simulink model "lump_model_v8"  (R2024b)
settings: Solver=FixedStepAuto  StartTime=0.0  StopTime=1079  FixedStep=0.001  RelTol=1e-3
model workspace (MAT data in the model file):
  A_busbar = 0.0015
  A_pack = 0.711626248
  C_nominal = 3
  I_max = 157.708978328
  P = 5
  S = 138
  SoC_initial = 0.78
  T_amb = 297.15
  W_max = 34
  busbar_CC_area = 0.000108
  busbar_Cp = 237
  busbar_length = 0.032
  busbar_mass = 0.01
  busbar_resistivity = 1.68e-08
  busbar_thermalcontact_resistance = 1
  cell_Cp = 1000
  cell_mass = 0.046
  h_busbar = 5
  h_pack = 5
(part 3 of 3)

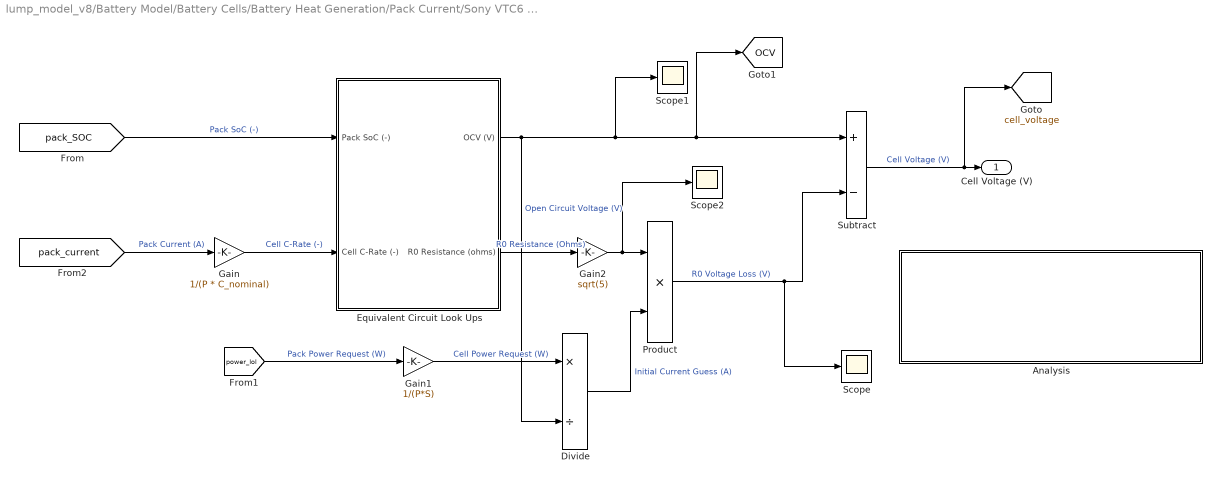
== system lump_model_v8/Battery Model/Battery Cells/Battery Heat Generation/Pack Current/Sony VTC6 Equivalent Circuit ==
  Analysis : Subsystem
  Divide : Product  Inputs=*/
  Equivalent Circuit Look Ups : Subsystem
  Gain : Gain  Gain=1/(P * C_nominal)
  Gain1 : Gain  Gain=1/(P*S)
  Gain2 : Gain  Gain=sqrt(5)
  Product : Product
  Scope : Scope
  Scope1 : Scope
  Scope2 : Scope
  Subtract : Sum  Inputs=+-
  Cell Voltage (V) : Outport
  tag scope: OCV=global, cell_voltage=global
  wires:
  [pack_SOC] -> Equivalent Circuit Look Ups/1(Pack SoC (-))  "Pack SoC (-)"
  Gain/1 -> Equivalent Circuit Look Ups/2(Cell C-Rate (-))  "Cell C-Rate (-)"
  Equivalent Circuit Look Ups/2(R0 Resistance (ohms)) -> Gain2/1  "R0 Resistance (Ohms)"
  Equivalent Circuit Look Ups/1(OCV (V)) -> Scope1/1, [OCV], Subtract/1, Divide/2  "Open Circuit Voltage (V)"
  Product/1 -> Scope/1, Subtract/2  "R0 Voltage Loss (V)"
  Subtract/1 -> [cell_voltage], Cell Voltage (V)/1  "Cell Voltage (V)"
  Divide/1 -> Product/2  "Initial Current Guess (A)"
  [power_lol] -> Gain1/1  "Pack Power Request (W)"
  Gain1/1 -> Divide/1  "Cell Power Request (W)"
  [pack_current] -> Gain/1  "Pack Current (A)"
  Gain2/1 -> Scope2/1, Product/1

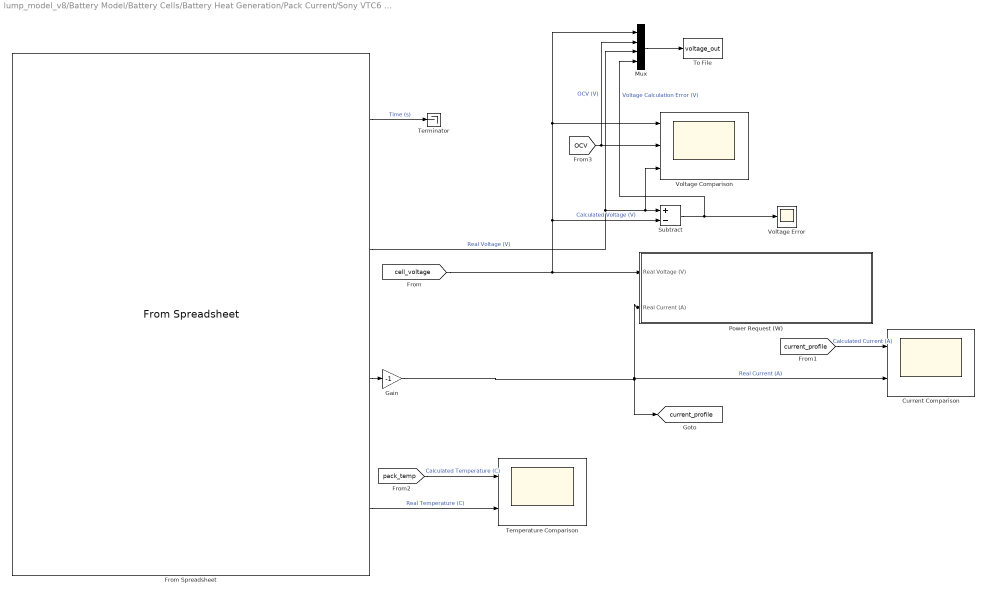
== system lump_model_v8/Battery Model/Battery Cells/Battery Heat Generation/Pack Current/Sony VTC6 Equivalent Circuit/Analysis ==
  Current Comparison : Scope  NumInputPorts=2
  From Spreadsheet : FromSpreadsheet  FileName=arbincomparisondata.xlsx  TreatFirstColumnAs=Data  SampleTime=0.003
  Gain : Gain  Gain=-1
  Mux : Mux
  Power Request (W) : Subsystem
  Subtract : Sum  Inputs=+-
  Temperature Comparison : Scope  NumInputPorts=2
  Terminator : Terminator
  To File : ToFile  Filename=voltage_out  MatrixName=voltage  SampleTime=0.01
  Voltage Comparison : Scope  NumInputPorts=3
  Voltage Error : Scope
  tag scope: current_profile=global
  wires:
  [cell_voltage] -> Power Request (W)/1(Real Voltage (V)), Subtract/2, Mux/1, Voltage Comparison/1  "Calculated Voltage (V)"
  [current_profile] -> Current Comparison/1  "Calculated Current (A)"
  [pack_temp] -> Temperature Comparison/1  "Calculated Temperature (C)"
  From Spreadsheet/2 -> Mux/3, Subtract/1, Voltage Comparison/3  "Real Voltage (V)"
  From Spreadsheet/3 -> Gain/1
  From Spreadsheet/4 -> Temperature Comparison/2  "Real Temperature (C)"
  From Spreadsheet/1 -> Terminator/1  "Time (s)"
  Gain/1 -> Current Comparison/2, Power Request (W)/2(Real Current (A)), [current_profile]  "Real Current (A)"
  Subtract/1 -> Mux/4, Voltage Error/1  "Voltage Calculation Error (V)"
  [OCV] -> Mux/2, Voltage Comparison/2  "OCV (V)"
  Mux/1 -> To File/1

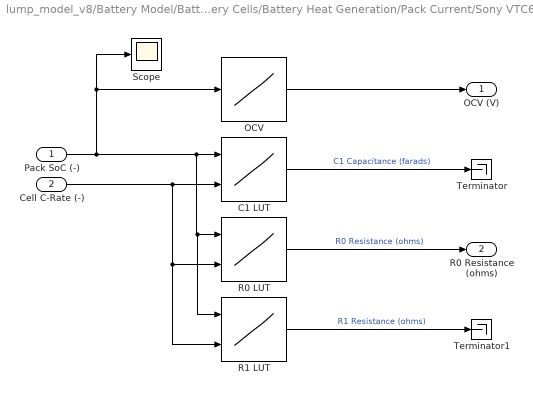
== system lump_model_v8/Battery Model/Battery Cells/Battery Heat Generation/Pack Current/Sony VTC6 Equivalent Circuit/Equivalent Circuit Look Ups ==
  Pack SoC (-) : Inport
  Cell C-Rate (-) : Inport  Port=2
  C1 LUT : Lookup_n-D  BreakpointsForDimension1=[0.1;0.2;0.3;0.4;0.5;0.6;0.7;0.8;0.9;1]  BreakpointsForDimension2=[-10;-5;-1;-0.333;0.333;1;2;3]  Table=[0.018906 0.021356 0.02305 0.022911 0.023301 0.023001 0.022654 0.019898;0.01868 0.020344 0.020909 0.020815 0.020944 0.020599 0.020712 0.017891;0.018453 0.019332 0.018859 0.023564 0.020028 0.019683 0.018901 0.017366;0.018226 0.019017 0.019644 0.020423 0.019635 0.019161 0.018682 0.01725;0.017999 0.018694 0.019687 0.020161 0.019897 0.01894 0.018442 0.01725;0.017916 0.018598 0.018989 0.01859 0.019505 0.018506 0.018289 0.017251;0.017743 0.018319 0.018291 0.022256 0.019767 0.018636 0.017788 0.017251;0.018183 0.018773 0.019295 0.021996 0.019898 0.019336 0.017286 0.017251;0.019549 0.020642 0.021608 0.025136 0.022253 0.020993 0.016785 0.017251;0.022703 0.024917 0.026536 0.026706 0.024609 0.02265 0.016283 0.017251]  ExtrapMethod=Clip  InternalRulePriority=Speed  RndMeth=Simplest
      settings: InputPortMap=u0,u1
  OCV : Lookup_n-D  NumberOfTableDimensions=1  BreakpointsForDimension1=[0.1;0.2;0.3;0.4;0.5;0.6;0.7;0.8;0.9;1]  BeginIndexSearchUsingPreviousIndexResult=on  Table=[3.227877;3.437376;3.537935;3.663634;3.755814;3.835423;3.940172;4.047017;4.097296;4.187904]  InternalRulePriority=Speed  RndMeth=Simplest
  R0 LUT : Lookup_n-D  BreakpointsForDimension1=[0.1;0.2;0.3;0.4;0.5;0.6;0.7;0.8;0.9;1]  BreakpointsForDimension2=[-10;-5;-1;-0.333;0.333;1;2;3]  Table=[0.018906 0.021356 0.02305 0.022911 0.023301 0.023001 0.022654 0.019898;0.01868 0.020344 0.020909 0.020815 0.020944 0.020599 0.020712 0.017891;0.018453 0.019332 0.018859 0.023564 0.020028 0.019683 0.018901 0.017366;0.018226 0.019017 0.019644 0.020423 0.019635 0.019161 0.018682 0.01725;0.017999 0.018694 0.019687 0.020161 0.019897 0.01894 0.018442 0.01725;0.017916 0.018598 0.018989 0.01859 0.019505 0.018506 0.018289 0.017251;0.017743 0.018319 0.018291 0.022256 0.019767 0.018636 0.017788 0.017251;0.018183 0.018773 0.019295 0.021996 0.019898 0.019336 0.017286 0.017251;0.019549 0.020642 0.021608 0.025136 0.022253 0.020993 0.016785 0.017251;0.022703 0.024917 0.026536 0.026706 0.024609 0.02265 0.016283 0.017251]  ExtrapMethod=Clip  InternalRulePriority=Speed  RndMeth=Simplest
      settings: InputPortMap=u0,u1
  R1 LUT : Lookup_n-D  BreakpointsForDimension1=[0.1;0.2;0.3;0.4;0.5;0.6;0.7;0.8;0.9;1]  BreakpointsForDimension2=[-10;-5;-1;-0.333;0.333;1;2;3]  Table=[0.018906 0.021356 0.02305 0.022911 0.023301 0.023001 0.022654 0.019898;0.01868 0.020344 0.020909 0.020815 0.020944 0.020599 0.020712 0.017891;0.018453 0.019332 0.018859 0.023564 0.020028 0.019683 0.018901 0.017366;0.018226 0.019017 0.019644 0.020423 0.019635 0.019161 0.018682 0.01725;0.017999 0.018694 0.019687 0.020161 0.019897 0.01894 0.018442 0.01725;0.017916 0.018598 0.018989 0.01859 0.019505 0.018506 0.018289 0.017251;0.017743 0.018319 0.018291 0.022256 0.019767 0.018636 0.017788 0.017251;0.018183 0.018773 0.019295 0.021996 0.019898 0.019336 0.017286 0.017251;0.019549 0.020642 0.021608 0.025136 0.022253 0.020993 0.016785 0.017251;0.022703 0.024917 0.026536 0.026706 0.024609 0.02265 0.016283 0.017251]  InternalRulePriority=Speed  RndMeth=Simplest
      settings: InputPortMap=u0,u1
  Scope : Scope
  Terminator : Terminator
  Terminator1 : Terminator
  OCV (V) : Outport
  R0 Resistance (ohms) : Outport  Port=2
  wires:
  Cell C-Rate (-)/1 -> R1 LUT/2, R0 LUT/2, C1 LUT/2
  Pack SoC (-)/1 -> Scope/1, OCV/1, C1 LUT/1, R1 LUT/1, R0 LUT/1
  C1 LUT/1 -> Terminator/1  "C1 Capacitance (farads)"
  R1 LUT/1 -> Terminator1/1  "R1 Resistance (ohms)"
  R0 LUT/1 -> R0 Resistance (ohms)/1  "R0 Resistance (ohms)"
  OCV/1 -> OCV (V)/1

== system lump_model_v8/Battery Model/Battery Cells/Battery Heat Generation/Pack Current/Sony VTC6 Equivalent Circuit/Analysis/Power Request (W) ==
  Real Voltage (V) : Inport
  Real Current (A) : Inport  Port=2
  Gain : Gain  Gain=S
  Product : Product
  tag scope: power_lol=global
  wires:
  Real Voltage (V)/1 -> Gain/1
  Gain/1 -> Product/1
  Real Current (A)/1 -> Product/2
  Product/1 -> [power_lol]
